simulink model "training_model_all"  (R2019b)
settings: Solver=VariableStepAuto  StartTime=0.0  StopTime=1500  RelTol=1e-3
values from neighbouring files (symbols this model uses):
  A = 0.5    [training.m]
  B = 0.5    [training.m]
  Belt_length = 0.5    [initialization.m]
  Distance_between = 0.05    [initialization.m]
  Entity_length = 0.05    [initialization.m]
  n = n+1    (= 2)    [training.m]
undefined symbols (not defined in the file or in its folder): m, T_product
libraries: simulink x6, sldelib x6, rllib x1
settings Model: Creator=Alexa  LastModifiedBy=Alexa

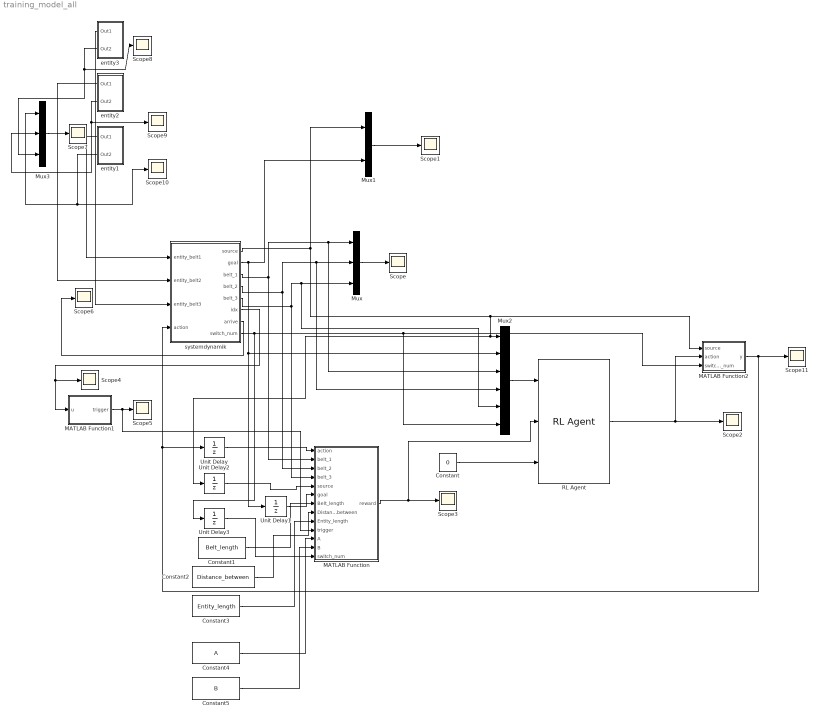
== system training_model_all ==
  Constant : Constant  Value=0
  Constant1 : Constant  Value=Belt_length
  Constant2 : Constant  Value=Distance_between
  Constant3 : Constant  Value=Entity_length
  Constant4 : Constant  Value=A
  Constant5 : Constant  Value=B
  MATLAB Function : MATLAB Function  TreatAsAtomicUnit=on
  MATLAB Function1 : MATLAB Function  TreatAsAtomicUnit=on
  MATLAB Function2 : MATLAB Function  TreatAsAtomicUnit=on
  Mux : Mux  Inputs=3
  Mux1 : Mux  Inputs=2
  Mux2 : Mux  Inputs=6
  Mux3 : Mux  Inputs=3
  RL Agent : rllib/RL Agent  Agent=agent  ProvideReward=on  ProvideIsDone=on  ProvideCumRwd=off  TreatAsDirectFeedthrough=on  CollectLoggedSignals=on  CollectModelStates=on
      settings: SourceProductName=Reinforcement Learning Toolbox
  Scope{,1..11} (12 alike) : Scope
  Unit Delay{,1..3} (4 alike) : UnitDelay  SampleTime=-1  HasFrameUpgradeWarning=on
  entity1 : Subsystem
  entity2 : Subsystem
  entity3 : Subsystem
  systemdynamik : Subsystem
  wires:
  Mux/1 -> Scope/1
  Mux1/1 -> Scope1/1
  Mux2/1 -> RL Agent/1
  Constant/1 -> RL Agent/3
  MATLAB Function/1(reward) -> Scope3/1, RL Agent/2
  systemdynamik/3(belt_1) -> MATLAB Function/2(belt_1), Mux2/3, Mux/1
  systemdynamik/5(belt_3) -> MATLAB Function/4(belt_3), Mux2/5, Mux/3
  systemdynamik/4(belt_2) -> MATLAB Function/3(belt_2), Mux2/4, Mux/2
  entity1/1(Out1) -> systemdynamik/1(entity_belt1)
  entity2/1(Out1) -> systemdynamik/2(entity_belt2)
  entity3/1(Out1) -> systemdynamik/3(entity_belt3)
  Constant1/1 -> MATLAB Function/7(Belt_length)
  Constant2/1 -> MATLAB Function/8(Distance_between)
  Constant3/1 -> MATLAB Function/9(Entity_length)
  systemdynamik/1(source) -> Unit Delay2/1, Mux2/1, MATLAB Function2/1(source), Mux1/1
  systemdynamik/2(goal) -> Mux1/2, Unit Delay1/1, Mux2/2
  Unit Delay/1 -> MATLAB Function/1(action)
  Unit Delay1/1 -> MATLAB Function/6(goal)
  Unit Delay2/1 -> MATLAB Function/5(source)
  systemdynamik/6(idx) -> Scope4/1, MATLAB Function1/1(u)
  MATLAB Function1/1(trigger) -> MATLAB Function/10(trigger), Scope5/1
  systemdynamik/7("arrive ") -> Scope6/1
  entity3/2(Out2) -> Mux3/3, Scope8/1
  entity2/2(Out2) -> Mux3/2, Scope9/1
  entity1/2(Out2) -> Scope10/1, Mux3/1
  RL Agent/1 -> Scope2/1, MATLAB Function2/2(action)
  MATLAB Function2/1(y) -> Scope11/1, Unit Delay/1, systemdynamik/4(action)
  Mux3/1 -> Scope7/1
  systemdynamik/8(switch_num) -> Mux2/6, MATLAB Function2/3(switch_num), Unit Delay3/1
  Unit Delay3/1 -> MATLAB Function/13(switch_num)
  Constant4/1 -> MATLAB Function/11(A)
  Constant5/1 -> MATLAB Function/12(B)

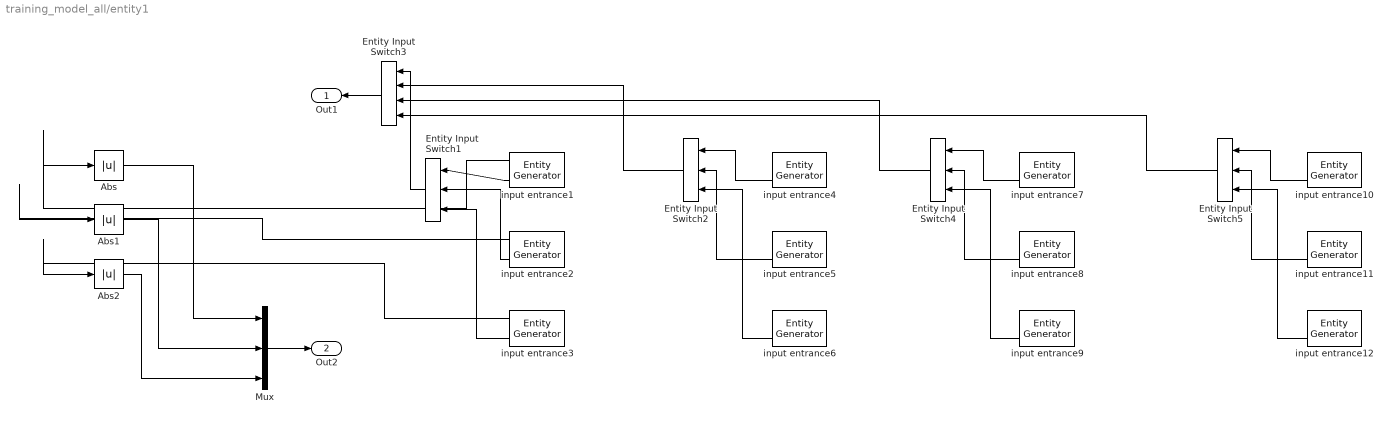
== system training_model_all/entity1 ==
  Abs : Abs
  Abs1 : Abs
  Abs2 : Abs
  Entity Input Switch{1..2,4..5} (4 alike) : EntityInputSwitch  InputPortMessageModes=m,m,m  OutputPortMessageModes=m  NumberInputPorts=3
      settings: InputPortMap=u1,u2,u3
  Entity Input Switch3 : EntityInputSwitch  InputPortMessageModes=m,m,m,m  OutputPortMessageModes=m  NumberInputPorts=4
      settings: InputPortMap=u1,u2,u3,u4
  Mux : Mux  Inputs=3
  input entrance1 : EntityGenerator  OutputPortMessageModes=n,m  TimeSource=MATLAB action  Period=T_product  IntergenerationTimeAction=|  AttributeName=source|goal|switch_num  AttributeInitialValue=1|1|1  NumberEntitiesDeparted=on  EntityType=Structured  EntityTypeName=Entity
      | % Pattern: Repeating Sequence
      | persistent idx1;
      | if isempty(idx1)
      |     idx1 = 1;
      | end
      | if idx1 > num
      |     dt = inf;
      | else
      |     dt = 3*T_interval;
      | end
      | idx1 = idx1 + 1;
      settings: OutputPortMap=o0,o3
  input entrance10 : EntityGenerator  OutputPortMessageModes=n,m  TimeSource=MATLAB action  Period=T_product  IntergenerationTimeAction=|  AttributeName=source|goal|switch_num  AttributeInitialValue=1|1|4  NumberEntitiesDeparted=on  EntityType=Structured  EntityTypeName=Entity
      | % Pattern: Repeating Sequence
      | persistent idx1;
      | if isempty(idx1)
      |     idx1 = 1;
      | end
      | if idx1==1
      |     dt = 900;
      | elseif idx1 > num
      |     dt = inf;
      | else
      |     dt = 3*T_interval;
      | end
      | idx1 = idx1 + 1;
      settings: OutputPortMap=o0,o3
  input entrance11 : EntityGenerator  OutputPortMessageModes=n,m  TimeSource=MATLAB action  Period=T_product  IntergenerationTimeAction=|  GenerateEntityAtSimulationStart=off  AttributeName=source|goal|switch_num  AttributeInitialValue=1|2|4  NumberEntitiesDeparted=on  EntityType=Structured  EntityTypeName=Entity
      | % Pattern: Repeating Sequence
      | persistent idx1;
      | if isempty(idx1)
      |     idx1 = 1;
      | end
      | if idx1==1
      |     dt =900+T_interval;
      | elseif idx1 > num
      |     dt = inf;
      | else
      |     dt = 3*T_interval;
      | end
      | idx1 = idx1 + 1;
      settings: OutputPortMap=o0,o3
  input entrance12 : EntityGenerator  OutputPortMessageModes=n,m  TimeSource=MATLAB action  Period=T_product  IntergenerationTimeAction=|  GenerateEntityAtSimulationStart=off  AttributeName=source|goal|switch_num  AttributeInitialValue=1|3|4  NumberEntitiesDeparted=on  EntityType=Structured  EntityTypeName=Entity
      | % Pattern: Repeating Sequence
      | persistent idx1;
      | if isempty(idx1)
      |     idx1 = 1;
      | end
      | if idx1==1
      |     dt = 900+2*T_interval;
      | elseif idx1 > num
      |     dt = inf;
      | else
      |     dt = 3*T_interval;
      | end
      | idx1 = idx1 + 1;
      settings: OutputPortMap=o0,o3
  input entrance2 : EntityGenerator  OutputPortMessageModes=n,m  TimeSource=MATLAB action  Period=T_product  IntergenerationTimeAction=|  GenerateEntityAtSimulationStart=off  AttributeName=source|goal|switch_num  AttributeInitialValue=1|2|1  NumberEntitiesDeparted=on  EntityType=Structured  EntityTypeName=Entity
      | % Pattern: Repeating Sequence
      | persistent idx1;
      | if isempty(idx1)
      |     idx1 = 1;
      | end
      | if idx1==1
      |     dt = T_interval;
      | elseif idx1 > num
      |     dt = inf;
      | else
      |     dt = 3*T_interval;
      | end
      | idx1 = idx1 + 1;
      settings: OutputPortMap=o0,o3
  input entrance3 : EntityGenerator  OutputPortMessageModes=n,m  TimeSource=MATLAB action  Period=T_product  IntergenerationTimeAction=|  GenerateEntityAtSimulationStart=off  AttributeName=source|goal|switch_num  AttributeInitialValue=1|3|1  NumberEntitiesDeparted=on  EntityType=Structured  EntityTypeName=Entity
      | % Pattern: Repeating Sequence
      | persistent idx1;
      | if isempty(idx1)
      |     idx1 = 1;
      | end
      | if idx1==1
      |     dt = 2*T_interval;
      | elseif idx1 > num
      |     dt = inf;
      | else
      |     dt = 3*T_interval;
      | end
      | idx1 = idx1 + 1;
      settings: OutputPortMap=o0,o3
  input entrance4 : EntityGenerator  OutputPortMessageModes=n,m  TimeSource=MATLAB action  Period=T_product  IntergenerationTimeAction=|  AttributeName=source|goal|switch_num  AttributeInitialValue=1|1|2  NumberEntitiesDeparted=on  EntityType=Structured  EntityTypeName=Entity
      | % Pattern: Repeating Sequence
      | persistent idx1;
      | if isempty(idx1)
      |     idx1 = 1;
      | end
      | if idx1==1
      |     dt = 300;
      | elseif idx1 > num
      |     dt = inf;
      | else
      |     dt = 3*T_interval;
      | end
      | idx1 = idx1 + 1;
      settings: OutputPortMap=o0,o3
  input entrance5 : EntityGenerator  OutputPortMessageModes=n,m  TimeSource=MATLAB action  Period=T_product  IntergenerationTimeAction=|  GenerateEntityAtSimulationStart=off  AttributeName=source|goal|switch_num  AttributeInitialValue=1|2|2  NumberEntitiesDeparted=on  EntityType=Structured  EntityTypeName=Entity
      | % Pattern: Repeating Sequence
      | persistent idx1;
      | if isempty(idx1)
      |     idx1 = 1;
      | end
      | if idx1==1
      |     dt =300+T_interval;
      | elseif idx1 > num
      |     dt = inf;
      | else
      |     dt = 3*T_interval;
      | end
      | idx1 = idx1 + 1;
      settings: OutputPortMap=o0,o3
  input entrance6 : EntityGenerator  OutputPortMessageModes=n,m  TimeSource=MATLAB action  Period=T_product  IntergenerationTimeAction=|  GenerateEntityAtSimulationStart=off  AttributeName=source|goal|switch_num  AttributeInitialValue=1|3|2  NumberEntitiesDeparted=on  EntityType=Structured  EntityTypeName=Entity
      | % Pattern: Repeating Sequence
      | persistent idx1;
      | if isempty(idx1)
      |     idx1 = 1;
      | end
      | if idx1==1
      |     dt = 300+2*T_interval;
      | elseif idx1 > num
      |     dt = inf;
      | else
      |     dt = 3*T_interval;
      | end
      | idx1 = idx1 + 1;
      settings: OutputPortMap=o0,o3
  input entrance7 : EntityGenerator  OutputPortMessageModes=n,m  TimeSource=MATLAB action  Period=T_product  IntergenerationTimeAction=|  AttributeName=source|goal|switch_num  AttributeInitialValue=1|1|3  NumberEntitiesDeparted=on  EntityType=Structured  EntityTypeName=Entity
      | % Pattern: Repeating Sequence
      | persistent idx1;
      | if isempty(idx1)
      |     idx1 = 1;
      | end
      | if idx1==1
      |     dt = 600;
      | elseif idx1 > num
      |     dt = inf;
      | else
      |     dt = 3*T_interval;
      | end
      | idx1 = idx1 + 1;
      settings: OutputPortMap=o0,o3
  input entrance8 : EntityGenerator  OutputPortMessageModes=n,m  TimeSource=MATLAB action  Period=T_product  IntergenerationTimeAction=|  GenerateEntityAtSimulationStart=off  AttributeName=source|goal|switch_num  AttributeInitialValue=1|2|3  NumberEntitiesDeparted=on  EntityType=Structured  EntityTypeName=Entity
      | % Pattern: Repeating Sequence
      | persistent idx1;
      | if isempty(idx1)
      |     idx1 = 1;
      | end
      | if idx1==1
      |     dt =600+T_interval;
      | elseif idx1 > num
      |     dt = inf;
      | else
      |     dt = 3*T_interval;
      | end
      | idx1 = idx1 + 1;
      settings: OutputPortMap=o0,o3
  input entrance9 : EntityGenerator  OutputPortMessageModes=n,m  TimeSource=MATLAB action  Period=T_product  IntergenerationTimeAction=|  GenerateEntityAtSimulationStart=off  AttributeName=source|goal|switch_num  AttributeInitialValue=1|3|3  NumberEntitiesDeparted=on  EntityType=Structured  EntityTypeName=Entity
      | % Pattern: Repeating Sequence
      | persistent idx1;
      | if isempty(idx1)
      |     idx1 = 1;
      | end
      | if idx1==1
      |     dt = 600+2*T_interval;
      | elseif idx1 > num
      |     dt = inf;
      | else
      |     dt = 3*T_interval;
      | end
      | idx1 = idx1 + 1;
      settings: OutputPortMap=o0,o3
  Out1 : Outport
  Out2 : Outport  Port=2
  wires:
  input entrance3/2 -> Entity Input Switch1/3
  input entrance1/2 -> Entity Input Switch1/1
  input entrance2/2 -> Entity Input Switch1/2
  Mux/1 -> Out2/1
  input entrance1/1 -> Abs/1
  input entrance2/1 -> Abs1/1
  input entrance3/1 -> Abs2/1
  Abs/1 -> Mux/1
  Abs1/1 -> Mux/2
  Abs2/1 -> Mux/3
  input entrance5/2 -> Entity Input Switch2/2
  input entrance4/2 -> Entity Input Switch2/1
  input entrance6/2 -> Entity Input Switch2/3
  Entity Input Switch3/1 -> Out1/1
  input entrance9/2 -> Entity Input Switch4/3
  input entrance7/2 -> Entity Input Switch4/1
  input entrance8/2 -> Entity Input Switch4/2
  input entrance11/2 -> Entity Input Switch5/2
  input entrance10/2 -> Entity Input Switch5/1
  input entrance12/2 -> Entity Input Switch5/3
  Entity Input Switch1/1 -> Entity Input Switch3/1
  Entity Input Switch2/1 -> Entity Input Switch3/2
  Entity Input Switch4/1 -> Entity Input Switch3/3
  Entity Input Switch5/1 -> Entity Input Switch3/4

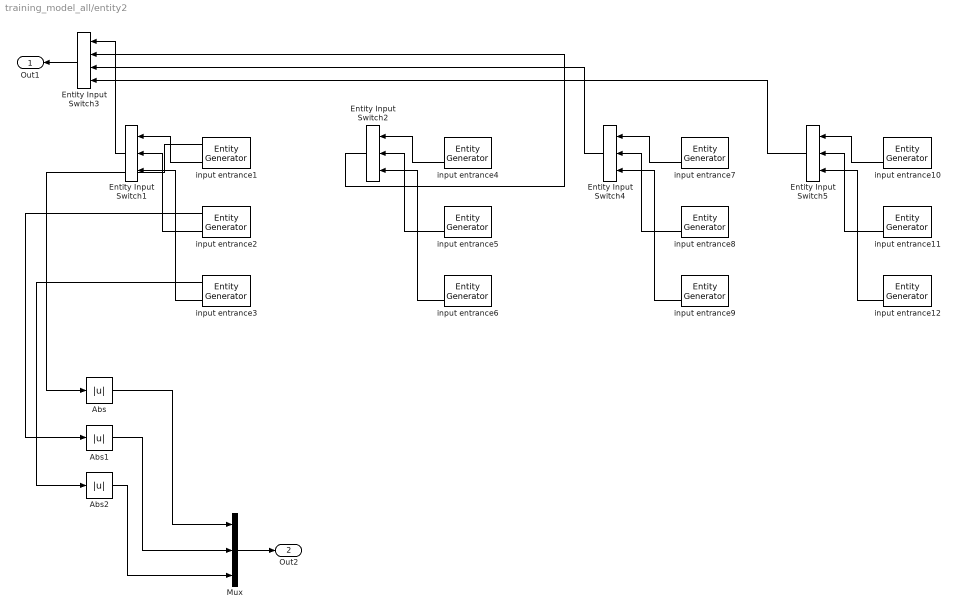
== system training_model_all/entity2 ==
  Abs : Abs
  Abs1 : Abs
  Abs2 : Abs
  Entity Input Switch{1..2,4..5} (4 alike) : EntityInputSwitch  InputPortMessageModes=m,m,m  OutputPortMessageModes=m  NumberInputPorts=3
      settings: InputPortMap=u1,u2,u3
  Entity Input Switch3 : EntityInputSwitch  InputPortMessageModes=m,m,m,m  OutputPortMessageModes=m  NumberInputPorts=4
      settings: InputPortMap=u1,u2,u3,u4
  Mux : Mux  Inputs=3
  input entrance1 : EntityGenerator  OutputPortMessageModes=n,m  TimeSource=MATLAB action  Period=T_product  IntergenerationTimeAction=|  GenerateEntityAtSimulationStart=off  AttributeName=source|goal|switch_num  AttributeInitialValue=2|1|1  NumberEntitiesDeparted=on  EntityType=Structured  EntityTypeName=Entity
      | % Pattern: Repeating Sequence
      | persistent idx1;
      | if isempty(idx1)
      |     idx1 = 1;
      | end
      | if idx1==1
      |     dt = 100;
      | elseif idx1 > num
      |     dt = inf;
      | else
      |     dt = 3*T_interval;
      | end
      | idx1 = idx1 + 1;
      settings: OutputPortMap=o0,o3
  input entrance10 : EntityGenerator  OutputPortMessageModes=n,m  TimeSource=MATLAB action  Period=T_product  IntergenerationTimeAction=|  GenerateEntityAtSimulationStart=off  AttributeName=source|goal|switch_num  AttributeInitialValue=2|1|4  NumberEntitiesDeparted=on  EntityType=Structured  EntityTypeName=Entity
      | % Pattern: Repeating Sequence
      | persistent idx1;
      | if isempty(idx1)
      |     idx1 = 1;
      | end
      | if idx1==1
      |     dt = 1000;
      | elseif idx1 > num
      |     dt = inf;
      | else
      |     dt = 3*T_interval;
      | end
      | idx1 = idx1 + 1;
      settings: OutputPortMap=o0,o3
  input entrance11 : EntityGenerator  OutputPortMessageModes=n,m  TimeSource=MATLAB action  Period=T_product  IntergenerationTimeAction=|  GenerateEntityAtSimulationStart=off  AttributeName=source|goal|switch_num  AttributeInitialValue=2|2|4  NumberEntitiesDeparted=on  EntityType=Structured  EntityTypeName=Entity
      | % Pattern: Repeating Sequence
      | persistent idx1;
      | if isempty(idx1)
      |     idx1 = 1;
      | end
      | if idx1==1
      |     dt = 1000+T_interval;
      | elseif idx1 > num
      |     dt = inf;
      | else
      |     dt = 3*T_interval;
      | end
      | idx1 = idx1 + 1;
      settings: OutputPortMap=o0,o3
  input entrance12 : EntityGenerator  OutputPortMessageModes=n,m  TimeSource=MATLAB action  Period=T_product  IntergenerationTimeAction=|  GenerateEntityAtSimulationStart=off  AttributeName=source|goal|switch_num  AttributeInitialValue=2|3|4  NumberEntitiesDeparted=on  EntityType=Structured  EntityTypeName=Entity
      | % Pattern: Repeating Sequence
      | persistent idx1;
      | if isempty(idx1)
      |     idx1 = 1;
      | end
      | if idx1==1
      |     dt = 1000+2*T_interval;
      | elseif idx1 > num
      |     dt = inf;
      | else
      |     dt = 3*T_interval;
      | end
      | idx1 = idx1 + 1;
      settings: OutputPortMap=o0,o3
  input entrance2 : EntityGenerator  OutputPortMessageModes=n,m  TimeSource=MATLAB action  Period=T_product  IntergenerationTimeAction=|  GenerateEntityAtSimulationStart=off  AttributeName=source|goal|switch_num  AttributeInitialValue=2|2|1  NumberEntitiesDeparted=on  EntityType=Structured  EntityTypeName=Entity
      | % Pattern: Repeating Sequence
      | persistent idx1;
      | if isempty(idx1)
      |     idx1 = 1;
      | end
      | if idx1==1
      |     dt = 100+T_interval;
      | elseif idx1 > num
      |     dt = inf;
      | else
      |     dt = 3*T_interval;
      | end
      | idx1 = idx1 + 1;
      settings: OutputPortMap=o0,o3
  input entrance3 : EntityGenerator  OutputPortMessageModes=n,m  TimeSource=MATLAB action  Period=T_product  IntergenerationTimeAction=|  GenerateEntityAtSimulationStart=off  AttributeName=source|goal|switch_num  AttributeInitialValue=2|3|1  NumberEntitiesDeparted=on  EntityType=Structured  EntityTypeName=Entity
      | % Pattern: Repeating Sequence
      | persistent idx1;
      | if isempty(idx1)
      |     idx1 = 1;
      | end
      | if idx1==1
      |     dt = 100+2*T_interval;
      | elseif idx1 > num
      |     dt = inf;
      | else
      |     dt = 3*T_interval;
      | end
      | idx1 = idx1 + 1;
      settings: OutputPortMap=o0,o3
  input entrance4 : EntityGenerator  OutputPortMessageModes=n,m  TimeSource=MATLAB action  Period=T_product  IntergenerationTimeAction=|  GenerateEntityAtSimulationStart=off  AttributeName=source|goal|switch_num  AttributeInitialValue=2|1|2  NumberEntitiesDeparted=on  EntityType=Structured  EntityTypeName=Entity
      | % Pattern: Repeating Sequence
      | persistent idx1;
      | if isempty(idx1)
      |     idx1 = 1;
      | end
      | if idx1==1
      |     dt = 400;
      | elseif idx1 > num
      |     dt = inf;
      | else
      |     dt = 3*T_interval;
      | end
      | idx1 = idx1 + 1;
      settings: OutputPortMap=o0,o3
  input entrance5 : EntityGenerator  OutputPortMessageModes=n,m  TimeSource=MATLAB action  Period=T_product  IntergenerationTimeAction=|  GenerateEntityAtSimulationStart=off  AttributeName=source|goal|switch_num  AttributeInitialValue=2|2|2  NumberEntitiesDeparted=on  EntityType=Structured  EntityTypeName=Entity
      | % Pattern: Repeating Sequence
      | persistent idx1;
      | if isempty(idx1)
      |     idx1 = 1;
      | end
      | if idx1==1
      |     dt = 400+T_interval;
      | elseif idx1 > num
      |     dt = inf;
      | else
      |     dt = 3*T_interval;
      | end
      | idx1 = idx1 + 1;
      settings: OutputPortMap=o0,o3
  input entrance6 : EntityGenerator  OutputPortMessageModes=n,m  TimeSource=MATLAB action  Period=T_product  IntergenerationTimeAction=|  GenerateEntityAtSimulationStart=off  AttributeName=source|goal|switch_num  AttributeInitialValue=2|3|2  NumberEntitiesDeparted=on  EntityType=Structured  EntityTypeName=Entity
      | % Pattern: Repeating Sequence
      | persistent idx1;
      | if isempty(idx1)
      |     idx1 = 1;
      | end
      | if idx1==1
      |     dt = 400+2*T_interval;
      | elseif idx1 > num
      |     dt = inf;
      | else
      |     dt = 3*T_interval;
      | end
      | idx1 = idx1 + 1;
      settings: OutputPortMap=o0,o3
  input entrance7 : EntityGenerator  OutputPortMessageModes=n,m  TimeSource=MATLAB action  Period=T_product  IntergenerationTimeAction=|  GenerateEntityAtSimulationStart=off  AttributeName=source|goal|switch_num  AttributeInitialValue=2|1|3  NumberEntitiesDeparted=on  EntityType=Structured  EntityTypeName=Entity
      | % Pattern: Repeating Sequence
      | persistent idx1;
      | if isempty(idx1)
      |     idx1 = 1;
      | end
      | if idx1==1
      |     dt = 700;
      | elseif idx1 > num
      |     dt = inf;
      | else
      |     dt = 3*T_interval;
      | end
      | idx1 = idx1 + 1;
      settings: OutputPortMap=o0,o3
  input entrance8 : EntityGenerator  OutputPortMessageModes=n,m  TimeSource=MATLAB action  Period=T_product  IntergenerationTimeAction=|  GenerateEntityAtSimulationStart=off  AttributeName=source|goal|switch_num  AttributeInitialValue=2|2|3  NumberEntitiesDeparted=on  EntityType=Structured  EntityTypeName=Entity
      | % Pattern: Repeating Sequence
      | persistent idx1;
      | if isempty(idx1)
      |     idx1 = 1;
      | end
      | if idx1==1
      |     dt = 700+T_interval;
      | elseif idx1 > num
      |     dt = inf;
      | else
      |     dt = 3*T_interval;
      | end
      | idx1 = idx1 + 1;
      settings: OutputPortMap=o0,o3
  input entrance9 : EntityGenerator  OutputPortMessageModes=n,m  TimeSource=MATLAB action  Period=T_product  IntergenerationTimeAction=|  GenerateEntityAtSimulationStart=off  AttributeName=source|goal|switch_num  AttributeInitialValue=2|3|3  NumberEntitiesDeparted=on  EntityType=Structured  EntityTypeName=Entity
      | % Pattern: Repeating Sequence
      | persistent idx1;
      | if isempty(idx1)
      |     idx1 = 1;
      | end
      | if idx1==1
      |     dt = 700+2*T_interval;
      | elseif idx1 > num
      |     dt = inf;
      | else
      |     dt = 3*T_interval;
      | end
      | idx1 = idx1 + 1;
      settings: OutputPortMap=o0,o3
  Out1 : Outport
  Out2 : Outport  Port=2
  wires:
  input entrance2/2 -> Entity Input Switch1/2
  input entrance1/2 -> Entity Input Switch1/1
  input entrance3/2 -> Entity Input Switch1/3
  Mux/1 -> Out2/1
  input entrance1/1 -> Abs/1
  input entrance2/1 -> Abs1/1
  input entrance3/1 -> Abs2/1
  Abs/1 -> Mux/1
  Abs1/1 -> Mux/2
  Abs2/1 -> Mux/3
  Entity Input Switch3/1 -> Out1/1
  input entrance6/2 -> Entity Input Switch2/3
  input entrance4/2 -> Entity Input Switch2/1
  input entrance5/2 -> Entity Input Switch2/2
  input entrance8/2 -> Entity Input Switch4/2
  input entrance7/2 -> Entity Input Switch4/1
  input entrance9/2 -> Entity Input Switch4/3
  input entrance12/2 -> Entity Input Switch5/3
  input entrance10/2 -> Entity Input Switch5/1
  input entrance11/2 -> Entity Input Switch5/2
  Entity Input Switch1/1 -> Entity Input Switch3/1
  Entity Input Switch2/1 -> Entity Input Switch3/2
  Entity Input Switch4/1 -> Entity Input Switch3/3
  Entity Input Switch5/1 -> Entity Input Switch3/4

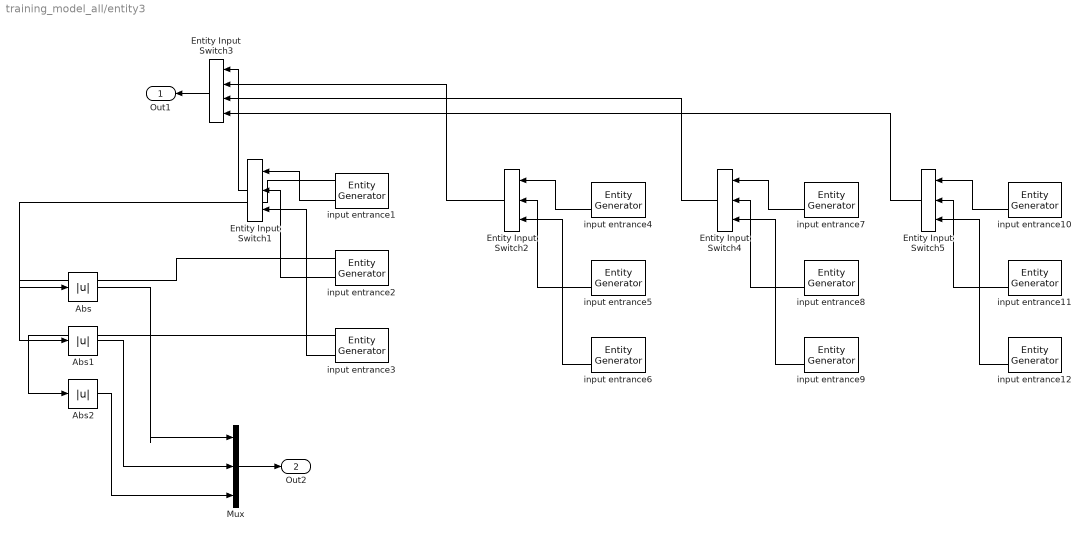
== system training_model_all/entity3 ==
  Abs : Abs
  Abs1 : Abs
  Abs2 : Abs
  Entity Input Switch{1..2,4..5} (4 alike) : EntityInputSwitch  InputPortMessageModes=m,m,m  OutputPortMessageModes=m  NumberInputPorts=3
      settings: InputPortMap=u1,u2,u3
  Entity Input Switch3 : EntityInputSwitch  InputPortMessageModes=m,m,m,m  OutputPortMessageModes=m  NumberInputPorts=4
      settings: InputPortMap=u1,u2,u3,u4
  Mux : Mux  Inputs=3
  input entrance1 : EntityGenerator  OutputPortMessageModes=n,m  TimeSource=MATLAB action  Period=T_product  IntergenerationTimeAction=|  GenerateEntityAtSimulationStart=off  AttributeName=source|goal|switch_num  AttributeInitialValue=3|1|1  NumberEntitiesDeparted=on  EntityType=Structured  EntityTypeName=Entity
      | % Pattern: Repeating Sequence
      | persistent idx1;
      | if isempty(idx1)
      |     idx1 = 1;
      | end
      | if idx1==1
      |     dt = 200;
      | elseif idx1 > num
      |     dt = inf;
      | else
      |     dt = 3*T_interval;
      | end
      | idx1 = idx1 + 1;
      settings: OutputPortMap=o0,o3
  input entrance10 : EntityGenerator  OutputPortMessageModes=n,m  TimeSource=MATLAB action  Period=T_product  IntergenerationTimeAction=|  GenerateEntityAtSimulationStart=off  AttributeName=source|goal|switch_num  AttributeInitialValue=3|1|4  NumberEntitiesDeparted=on  EntityType=Structured  EntityTypeName=Entity
      | % Pattern: Repeating Sequence
      | persistent idx1;
      | if isempty(idx1)
      |     idx1 = 1;
      | end
      | if idx1==1
      |     dt = 1100;
      | elseif idx1 > num
      |     dt = inf;
      | else
      |     dt = 3*T_interval;
      | end
      | idx1 = idx1 + 1;
      settings: OutputPortMap=o0,o3
  input entrance11 : EntityGenerator  OutputPortMessageModes=n,m  TimeSource=MATLAB action  Period=T_product  IntergenerationTimeAction=|  GenerateEntityAtSimulationStart=off  AttributeName=source|goal|switch_num  AttributeInitialValue=3|2|4  NumberEntitiesDeparted=on  EntityType=Structured  EntityTypeName=Entity
      | % Pattern: Repeating Sequence
      | persistent idx1;
      | if isempty(idx1)
      |     idx1 = 1;
      | end
      | if idx1==1
      |     dt = 1100+T_interval;
      | elseif idx1 > num
      |     dt = inf;
      | else
      |     dt = 3*T_interval;
      | end
      | idx1 = idx1 + 1;
      settings: OutputPortMap=o0,o3
  input entrance12 : EntityGenerator  OutputPortMessageModes=n,m  TimeSource=MATLAB action  Period=T_product  IntergenerationTimeAction=|  GenerateEntityAtSimulationStart=off  AttributeName=source|goal|switch_num  AttributeInitialValue=3|3|4  NumberEntitiesDeparted=on  EntityType=Structured  EntityTypeName=Entity
      | % Pattern: Repeating Sequence
      | persistent idx1;
      | if isempty(idx1)
      |     idx1 = 1;
      | end
      | if idx1==1
      |     dt = 1100+2*T_interval;
      | elseif idx1 > num
      |     dt = inf;
      | else
      |     dt = 3*T_interval;
      | end
      | idx1 = idx1 + 1;
      settings: OutputPortMap=o0,o3
  input entrance2 : EntityGenerator  OutputPortMessageModes=n,m  TimeSource=MATLAB action  Period=T_product  IntergenerationTimeAction=|  GenerateEntityAtSimulationStart=off  AttributeName=source|goal|switch_num  AttributeInitialValue=3|2|1  NumberEntitiesDeparted=on  EntityType=Structured  EntityTypeName=Entity
      | % Pattern: Repeating Sequence
      | persistent idx1;
      | if isempty(idx1)
      |     idx1 = 1;
      | end
      | if idx1==1
      |     dt = 200+T_interval;
      | elseif idx1 > num
      |     dt = inf;
      | else
      |     dt = 3*T_interval;
      | end
      | idx1 = idx1 + 1;
      settings: OutputPortMap=o0,o3
  input entrance3 : EntityGenerator  OutputPortMessageModes=n,m  TimeSource=MATLAB action  Period=T_product  IntergenerationTimeAction=|  GenerateEntityAtSimulationStart=off  AttributeName=source|goal|switch_num  AttributeInitialValue=3|3|1  NumberEntitiesDeparted=on  EntityType=Structured  EntityTypeName=Entity
      | % Pattern: Repeating Sequence
      | persistent idx1;
      | if isempty(idx1)
      |     idx1 = 1;
      | end
      | if idx1==1
      |     dt = 200+2*T_interval;
      | elseif idx1 > num
      |     dt = inf;
      | else
      |     dt = 3*T_interval;
      | end
      | idx1 = idx1 + 1;
      settings: OutputPortMap=o0,o3
  input entrance4 : EntityGenerator  OutputPortMessageModes=n,m  TimeSource=MATLAB action  Period=T_product  IntergenerationTimeAction=|  GenerateEntityAtSimulationStart=off  AttributeName=source|goal|switch_num  AttributeInitialValue=3|1|2  NumberEntitiesDeparted=on  EntityType=Structured  EntityTypeName=Entity
      | % Pattern: Repeating Sequence
      | persistent idx1;
      | if isempty(idx1)
      |     idx1 = 1;
      | end
      | if idx1==1
      |     dt = 500;
      | elseif idx1 > num
      |     dt = inf;
      | else
      |     dt = 3*T_interval;
      | end
      | idx1 = idx1 + 1;
      settings: OutputPortMap=o0,o3
  input entrance5 : EntityGenerator  OutputPortMessageModes=n,m  TimeSource=MATLAB action  Period=T_product  IntergenerationTimeAction=|  GenerateEntityAtSimulationStart=off  AttributeName=source|goal|switch_num  AttributeInitialValue=3|2|2  NumberEntitiesDeparted=on  EntityType=Structured  EntityTypeName=Entity
      | % Pattern: Repeating Sequence
      | persistent idx1;
      | if isempty(idx1)
      |     idx1 = 1;
      | end
      | if idx1==1
      |     dt = 500+T_interval;
      | elseif idx1 > num
      |     dt = inf;
      | else
      |     dt = 3*T_interval;
      | end
      | idx1 = idx1 + 1;
      settings: OutputPortMap=o0,o3
  input entrance6 : EntityGenerator  OutputPortMessageModes=n,m  TimeSource=MATLAB action  Period=T_product  IntergenerationTimeAction=|  GenerateEntityAtSimulationStart=off  AttributeName=source|goal|switch_num  AttributeInitialValue=3|3|2  NumberEntitiesDeparted=on  EntityType=Structured  EntityTypeName=Entity
      | % Pattern: Repeating Sequence
      | persistent idx1;
      | if isempty(idx1)
      |     idx1 = 1;
      | end
      | if idx1==1
      |     dt = 500+2*T_interval;
      | elseif idx1 > num
      |     dt = inf;
      | else
      |     dt = 3*T_interval;
      | end
      | idx1 = idx1 + 1;
      settings: OutputPortMap=o0,o3
  input entrance7 : EntityGenerator  OutputPortMessageModes=n,m  TimeSource=MATLAB action  Period=T_product  IntergenerationTimeAction=|  GenerateEntityAtSimulationStart=off  AttributeName=source|goal|switch_num  AttributeInitialValue=3|1|3  NumberEntitiesDeparted=on  EntityType=Structured  EntityTypeName=Entity
      | % Pattern: Repeating Sequence
      | persistent idx1;
      | if isempty(idx1)
      |     idx1 = 1;
      | end
      | if idx1==1
      |     dt = 800;
      | elseif idx1 > num
      |     dt = inf;
      | else
      |     dt = 3*T_interval;
      | end
      | idx1 = idx1 + 1;
      settings: OutputPortMap=o0,o3
  input entrance8 : EntityGenerator  OutputPortMessageModes=n,m  TimeSource=MATLAB action  Period=T_product  IntergenerationTimeAction=|  GenerateEntityAtSimulationStart=off  AttributeName=source|goal|switch_num  AttributeInitialValue=3|2|3  NumberEntitiesDeparted=on  EntityType=Structured  EntityTypeName=Entity
      | % Pattern: Repeating Sequence
      | persistent idx1;
      | if isempty(idx1)
      |     idx1 = 1;
      | end
      | if idx1==1
      |     dt = 800+T_interval;
      | elseif idx1 > num
      |     dt = inf;
      | else
      |     dt = 3*T_interval;
      | end
      | idx1 = idx1 + 1;
      settings: OutputPortMap=o0,o3
  input entrance9 : EntityGenerator  OutputPortMessageModes=n,m  TimeSource=MATLAB action  Period=T_product  IntergenerationTimeAction=|  GenerateEntityAtSimulationStart=off  AttributeName=source|goal|switch_num  AttributeInitialValue=3|3|3  NumberEntitiesDeparted=on  EntityType=Structured  EntityTypeName=Entity
      | % Pattern: Repeating Sequence
      | persistent idx1;
      | if isempty(idx1)
      |     idx1 = 1;
      | end
      | if idx1==1
      |     dt = 800+2*T_interval;
      | elseif idx1 > num
      |     dt = inf;
      | else
      |     dt = 3*T_interval;
      | end
      | idx1 = idx1 + 1;
      settings: OutputPortMap=o0,o3
  Out1 : Outport
  Out2 : Outport  Port=2
  wires:
  input entrance3/2 -> Entity Input Switch1/3
  input entrance1/2 -> Entity Input Switch1/1
  input entrance2/2 -> Entity Input Switch1/2
  input entrance1/1 -> Abs/1
  input entrance2/1 -> Abs1/1
  input entrance3/1 -> Abs2/1
  Abs/1 -> Mux/1
  Abs1/1 -> Mux/2
  Abs2/1 -> Mux/3
  Mux/1 -> Out2/1
  Entity Input Switch3/1 -> Out1/1
  input entrance5/2 -> Entity Input Switch2/2
  input entrance4/2 -> Entity Input Switch2/1
  input entrance6/2 -> Entity Input Switch2/3
  input entrance9/2 -> Entity Input Switch4/3
  input entrance7/2 -> Entity Input Switch4/1
  input entrance8/2 -> Entity Input Switch4/2
  input entrance11/2 -> Entity Input Switch5/2
  input entrance10/2 -> Entity Input Switch5/1
  input entrance12/2 -> Entity Input Switch5/3
  Entity Input Switch1/1 -> Entity Input Switch3/1
  Entity Input Switch2/1 -> Entity Input Switch3/2
  Entity Input Switch4/1 -> Entity Input Switch3/3
  Entity Input Switch5/1 -> Entity Input Switch3/4

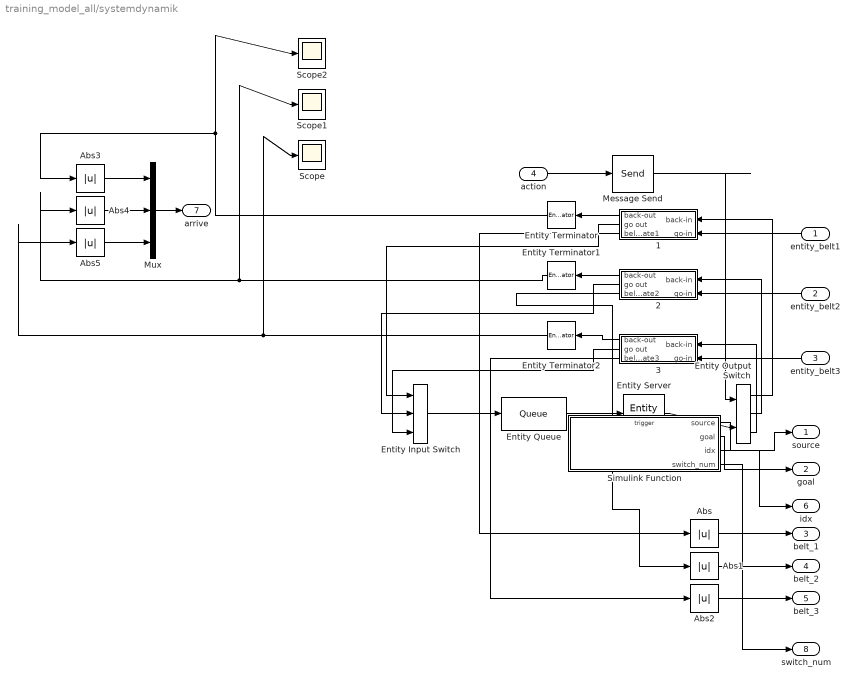
== system training_model_all/systemdynamik ==
  entity_belt1 : Inport
  entity_belt2 : Inport  Port=2
  entity_belt3 : Inport  Port=3
  action : Inport  Port=4
  "1 " : Subsystem
  "2 " : Subsystem
  "3 " : Subsystem
  Abs{,1..5} (6 alike) : Abs
  Entity Input Switch : EntityInputSwitch  InputPortMessageModes=m,m,m  OutputPortMessageModes=m  NumberInputPorts=3
      settings: InputPortMap=u1,u2,u3
  Entity Output Switch : EntityOutputSwitch  InputPortMessageModes=m,m  OutputPortMessageModes=m,m,m  NumberOutputPorts=3  SwitchingCriterion=From control port  SwitchAttributeName=Attribute1
      settings: InputPortMap=u0,u1  OutputPortMap=o0,o1,o2
  Entity Queue : Queue  InputPortMessageModes=m  OutputPortMessageModes=m  Capacity=1
  Entity Server : EntityServer  InputPortMessageModes=m  OutputPortMessageModes=m  Capacity=1  ServiceTimeValue=T_switch  EntryAction=|
      | persistent idx
      | if isempty(idx)
      |     idx=1;
      | end
      | getattribute(entity.source,entity.goal,idx,entity.switch_num);
      | idx=idx+1;
  Entity Terminator : EntityTerminator  InputPortMessageModes=m  NumberEntitiesArrived=on
      settings: OutputPortMap=o0
  Entity Terminator1 : EntityTerminator  InputPortMessageModes=m  NumberEntitiesArrived=on
      settings: OutputPortMap=o0
  Entity Terminator2 : EntityTerminator  InputPortMessageModes=m  NumberEntitiesArrived=on
      settings: OutputPortMap=o0
  Message Send : Send  OutputPortMessageModes=m
  Mux : Mux  Inputs=3
  Scope : Scope
  Scope1 : Scope
  Scope2 : Scope
  Simulink Function : Subsystem  TreatAsAtomicUnit=on
  source : Outport
  goal : Outport  Port=2
  belt_1 : Outport  Port=3
  belt_2 : Outport  Port=4
  belt_3 : Outport  Port=5
  idx : Outport  Port=6
  "arrive " : Outport  Port=7
  switch_num : Outport  Port=8
  wires:
  Entity Output Switch/3 -> "3 "/1(back-in)
  Entity Input Switch/1 -> Entity Queue/1
  "3 "/2(go out) -> Entity Input Switch/3
  "3 "/3(beltstate3) -> Abs2/1
  "1 "/2(go out) -> Entity Input Switch/1
  "1 "/1(back-out) -> Entity Terminator/1
  Entity Output Switch/2 -> "2 "/1(back-in)
  Entity Queue/1 -> Entity Server/1
  Entity Output Switch/1 -> "1 "/1(back-in)
  "2 "/2(go out) -> Entity Input Switch/2
  Entity Server/1 -> Entity Output Switch/2
  "2 "/1(back-out) -> Entity Terminator1/1
  "3 "/1(back-out) -> Entity Terminator2/1
  "2 "/3(beltstate2) -> Abs1/1
  "1 "/3(beltstate1) -> Abs/1
  entity_belt1/1 -> "1 "/2(go-in)
  entity_belt2/1 -> "2 "/2(go-in)
  Abs/1 -> belt_1/1
  Abs2/1 -> belt_3/1
  entity_belt3/1 -> "3 "/2(go-in)
  Simulink Function/1(source) -> source/1
  Simulink Function/2(goal) -> goal/1
  Abs1/1 -> belt_2/1
  Message Send/1 -> Entity Output Switch/1
  Simulink Function/3(idx) -> idx/1
  Abs4/1 -> Mux/2
  Abs5/1 -> Mux/3
  Abs3/1 -> Mux/1
  Entity Terminator/1 -> Scope2/1, Abs3/1
  Entity Terminator1/1 -> Abs4/1, Scope1/1
  Entity Terminator2/1 -> Scope/1, Abs5/1
  Mux/1 -> "arrive "/1
  action/1 -> Message Send/1
  Simulink Function/4(switch_num) -> switch_num/1

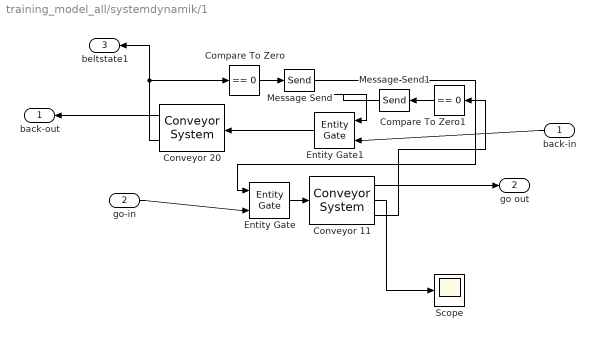
== system training_model_all/systemdynamik/1  ==
  back-in : Inport
  go-in : Inport  Port=2
  Compare To Zero : simulink/Logic and Bit Operations/Compare To Zero  relop===  OutDataTypeStr=boolean
  Compare To Zero1 : simulink/Logic and Bit Operations/Compare To Zero  relop===  OutDataTypeStr=boolean
  Conveyor 11 : sldelib/Conveyor System  mConveyorLength=4*Belt_length  mConveyorSpeedSource=Dialog  mConveyorSpeed=V_belt  mInitialConveyorSpeed=1000  mMinDisBetEntity=Distance_between  mEntityLengthSource=Dialog  mEntityLength=Entity_length  mEntityLengthAttrName=Length  mOutputBlockedOpt=Pause  mErrorUponFullOpt=on  mNumEntitiesDepOpt=on  mNumEntitiesInBlockOpt=on  mEntityPendingOpt=off  mNumExtractedFromBlockOpt=off  mConveyorSpeedOpt=off
      settings: SourceProductName=SimEvents  SourceProductBaseCode=SE
  Conveyor 20 : sldelib/Conveyor System  mConveyorLength=4*Belt_length  mConveyorSpeedSource=Dialog  mConveyorSpeed=V_belt  mInitialConveyorSpeed=1000  mMinDisBetEntity=Distance_between  mEntityLengthSource=Dialog  mEntityLength=Entity_length  mEntityLengthAttrName=Length  mOutputBlockedOpt=Pause  mErrorUponFullOpt=on  mNumEntitiesDepOpt=off  mNumEntitiesInBlockOpt=on  mEntityPendingOpt=off  mNumExtractedFromBlockOpt=off  mConveyorSpeedOpt=off
      settings: SourceProductName=SimEvents  SourceProductBaseCode=SE
  Entity Gate : EntityGate  InputPortMessageModes=m,m  OutputPortMessageModes=m
  Entity Gate1 : EntityGate  InputPortMessageModes=m,m  OutputPortMessageModes=m
  Message Send : Send  OutputPortMessageModes=m
  Message Send1 : Send  OutputPortMessageModes=m
  Scope : Scope
  back-out : Outport
  go out : Outport  Port=2
  beltstate1 : Outport  Port=3
  wires:
  go-in/1 -> Entity Gate/2
  Conveyor 20/1 -> back-out/1
  back-in/1 -> Entity Gate1/2
  Compare To Zero1/1 -> Message Send1/1
  Message Send1/1 -> Entity Gate1/1
  Entity Gate1/1 -> Conveyor 20/1
  Conveyor 11/1 -> go out/1
  Entity Gate/1 -> Conveyor 11/1
  Compare To Zero/1 -> Message Send/1
  Message Send/1 -> Entity Gate/1
  Conveyor 11/3 -> Compare To Zero1/1
  Conveyor 20/2 -> Compare To Zero/1, beltstate1/1
  Conveyor 11/2 -> Scope/1

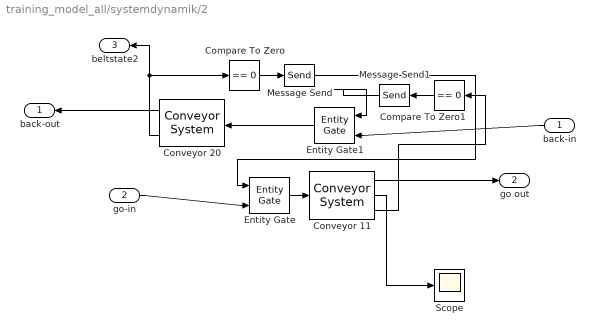
== system training_model_all/systemdynamik/2  ==
  back-in : Inport
  go-in : Inport  Port=2
  Compare To Zero : simulink/Logic and Bit Operations/Compare To Zero  relop===  OutDataTypeStr=boolean
  Compare To Zero1 : simulink/Logic and Bit Operations/Compare To Zero  relop===  OutDataTypeStr=boolean
  Conveyor 11 : sldelib/Conveyor System  mConveyorLength=4*Belt_length  mConveyorSpeedSource=Dialog  mConveyorSpeed=V_belt  mInitialConveyorSpeed=1000  mMinDisBetEntity=Distance_between  mEntityLengthSource=Dialog  mEntityLength=Entity_length  mEntityLengthAttrName=Length  mOutputBlockedOpt=Pause  mErrorUponFullOpt=on  mNumEntitiesDepOpt=on  mNumEntitiesInBlockOpt=on  mEntityPendingOpt=off  mNumExtractedFromBlockOpt=off  mConveyorSpeedOpt=off
      settings: SourceProductName=SimEvents  SourceProductBaseCode=SE
  Conveyor 20 : sldelib/Conveyor System  mConveyorLength=4*Belt_length  mConveyorSpeedSource=Dialog  mConveyorSpeed=V_belt  mInitialConveyorSpeed=1000  mMinDisBetEntity=Distance_between  mEntityLengthSource=Dialog  mEntityLength=Entity_length  mEntityLengthAttrName=Length  mOutputBlockedOpt=Pause  mErrorUponFullOpt=on  mNumEntitiesDepOpt=off  mNumEntitiesInBlockOpt=on  mEntityPendingOpt=off  mNumExtractedFromBlockOpt=off  mConveyorSpeedOpt=off
      settings: SourceProductName=SimEvents  SourceProductBaseCode=SE
  Entity Gate : EntityGate  InputPortMessageModes=m,m  OutputPortMessageModes=m
  Entity Gate1 : EntityGate  InputPortMessageModes=m,m  OutputPortMessageModes=m
  Message Send : Send  OutputPortMessageModes=m
  Message Send1 : Send  OutputPortMessageModes=m
  Scope : Scope
  back-out : Outport
  go out : Outport  Port=2
  beltstate2 : Outport  Port=3
  wires:
  Conveyor 11/2 -> Scope/1
  Conveyor 20/2 -> beltstate2/1, Compare To Zero/1
  Conveyor 11/3 -> Compare To Zero1/1
  Message Send/1 -> Entity Gate/1
  Compare To Zero/1 -> Message Send/1
  Entity Gate/1 -> Conveyor 11/1
  Conveyor 11/1 -> go out/1
  Entity Gate1/1 -> Conveyor 20/1
  Message Send1/1 -> Entity Gate1/1
  Compare To Zero1/1 -> Message Send1/1
  back-in/1 -> Entity Gate1/2
  Conveyor 20/1 -> back-out/1
  go-in/1 -> Entity Gate/2

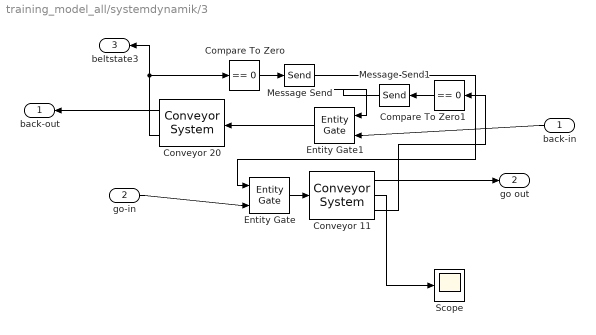
== system training_model_all/systemdynamik/3  ==
  back-in : Inport
  go-in : Inport  Port=2
  Compare To Zero : simulink/Logic and Bit Operations/Compare To Zero  relop===  OutDataTypeStr=boolean
  Compare To Zero1 : simulink/Logic and Bit Operations/Compare To Zero  relop===  OutDataTypeStr=boolean
  Conveyor 11 : sldelib/Conveyor System  mConveyorLength=Belt_length  mConveyorSpeedSource=Dialog  mConveyorSpeed=V_belt  mInitialConveyorSpeed=1000  mMinDisBetEntity=Distance_between  mEntityLengthSource=Dialog  mEntityLength=Entity_length  mEntityLengthAttrName=Length  mOutputBlockedOpt=Pause  mErrorUponFullOpt=on  mNumEntitiesDepOpt=on  mNumEntitiesInBlockOpt=on  mEntityPendingOpt=off  mNumExtractedFromBlockOpt=off  mConveyorSpeedOpt=off
      settings: SourceProductName=SimEvents  SourceProductBaseCode=SE
  Conveyor 20 : sldelib/Conveyor System  mConveyorLength=Belt_length  mConveyorSpeedSource=Dialog  mConveyorSpeed=V_belt  mInitialConveyorSpeed=1000  mMinDisBetEntity=Distance_between  mEntityLengthSource=Dialog  mEntityLength=Entity_length  mEntityLengthAttrName=Length  mOutputBlockedOpt=Pause  mErrorUponFullOpt=on  mNumEntitiesDepOpt=off  mNumEntitiesInBlockOpt=on  mEntityPendingOpt=off  mNumExtractedFromBlockOpt=off  mConveyorSpeedOpt=off
      settings: SourceProductName=SimEvents  SourceProductBaseCode=SE
  Entity Gate : EntityGate  InputPortMessageModes=m,m  OutputPortMessageModes=m
  Entity Gate1 : EntityGate  InputPortMessageModes=m,m  OutputPortMessageModes=m
  Message Send : Send  OutputPortMessageModes=m
  Message Send1 : Send  OutputPortMessageModes=m
  Scope : Scope
  back-out : Outport
  go out : Outport  Port=2
  beltstate3 : Outport  Port=3
  wires:
  Conveyor 11/2 -> Scope/1
  Conveyor 20/2 -> beltstate3/1, Compare To Zero/1
  Conveyor 11/3 -> Compare To Zero1/1
  Message Send/1 -> Entity Gate/1
  Compare To Zero/1 -> Message Send/1
  Entity Gate/1 -> Conveyor 11/1
  Conveyor 11/1 -> go out/1
  Entity Gate1/1 -> Conveyor 20/1
  Message Send1/1 -> Entity Gate1/1
  Compare To Zero1/1 -> Message Send1/1
  back-in/1 -> Entity Gate1/2
  Conveyor 20/1 -> back-out/1
  go-in/1 -> Entity Gate/2

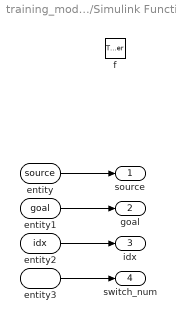
== system training_model_all/systemdynamik/Simulink Function ==
  f : TriggerPort  TriggerType=function-call  IsSimulinkFunction=on  FunctionName=getattribute  VariantControl=(inherit)
  entity : ArgIn  DisableCoverage=on  ArgumentName=source
  entity1 : ArgIn  DisableCoverage=on  Port=2  ArgumentName=goal
  entity2 : ArgIn  DisableCoverage=on  Port=3  ArgumentName=idx
  entity3 : ArgIn  DisableCoverage=on  Port=4  ArgumentName=switch_num
  source : Outport
  goal : Outport  Port=2
  idx : Outport  Port=3
  switch_num : Outport  Port=4
  wires:
  entity/1 -> source/1
  entity1/1 -> goal/1
  entity2/1 -> idx/1
  entity3/1 -> switch_num/1

== matlab function training_model_all/MATLAB Function1 ==
  data: u input; trigger output
function trigger= fcn(u)
persistent idx_0
if isempty(idx_0)
    idx_0=1;
end
if u==0
    trigger=0;
elseif u==idx_0
    trigger=1;
    idx_0=idx_0+1;
else
    trigger=0;
end

== matlab function training_model_all/MATLAB Function ==
  data: action input; reward output; belt_1 input; belt_2 input; belt_3 input; source input; goal input; Belt_length input; Distance_between input; Entity_length input; trigger input; A input; B input; switch_num input
function reward = fcn(action,belt_1,belt_2,belt_3,source,goal,Belt_length,Distance_between,Entity_length,trigger,A,B,switch_num)
%persistent source_default
%persistent goal_default

%source_default=source;
%goal_default=goal;
if switch_num==3
    Distance_reward=-[15,25,20;15,25,25;15,5,35]; %switch_3
elseif switch_num==2
    Distance_reward=-[20,10,20;20,10,20;20,20,10]; %switch_2
elseif switch_num==1
    Distance_reward=-[25,15;20,15;35,15]; %switch_1
else
    Distance_reward=-[35,15,15;15,35,15;35,25,15]; %switch_4
end
if source==1
    num_variance=abs(belt_2-belt_3);
elseif source==2
    num_variance=abs(belt_1-belt_3);
else
    num_variance=abs(belt_1-belt_2);
end
%if action==source&&source~=0||belt_1+belt_2+belt_3==0
% if belt_1+belt_2+belt_3==0
%     punish=1;
% else
%     punish=0;
% end
if switch_num==4
    if (goal==1&&action==2)||(goal==2&&action==1) % if reach goal give extra reward
        reach_goal=1;
    else
        reach_goal=0;
    end
elseif switch_num==3
    if (goal==1&&action==3)||(goal==3&&action==2) % if reach goal give extra reward
        reach_goal=1;
    else
        reach_goal=0;
    end
elseif switch_num==1
    if goal==2&&action==1 % if reach goal give extra reward
        reach_goal=1;
    else
        reach_goal=0;
    end
else
    reach_goal=0;
end
if source==0&&goal==0
    reward=0;
else
    if trigger==1
        reward=A*Distance_reward(goal,action)+B*(-num_variance)+5*reach_goal;
    else
        reward=0;
    end
%     reward = A*(Distance_reward(goal,action)-min(min(Distance_reward)))/(max(max(Distance_reward))-min(min(Distance_reward)))...
%             +B*((-num_variance)+4*Belt_length/(Distance_between+Entity_length))/(4*Belt_length/(Distance_between+Entity_length))...
%             +(-inf)*punish;

end

== matlab function training_model_all/MATLAB Function2 ==
  data: source input; y output; action input; switch_num input
function y = fcn(source,action,switch_num)
% switch_1
if switch_num==1
    if source==1
        y=2;
    elseif source==2
        y=1;
    else
        if action==1
            y=1;
        else
            y=2;
        end
    end
else
    if source==1
        if action==1
            y=2;
        else
            y=3;
        end
    elseif source==2
        if action==1
            y=1;
        else
            y=3;
        end
    elseif source==3
        if action==1
            y=1;
        else
            y=2;
        end
    else
        y=1;
    end
end
%% switch_1
% if source==1
%     y=2;
% elseif source==2
%     y=1;
% else
%     if action==1
%         y=1;
%     else
%         y=2;
%     end
% end
end
